simulink model "SchemaNO_DIS"  (R2020b)
settings: Solver=VariableStepAuto  StartTime=0.0  StopTime=20.0  RelTol=1e-3
undefined symbols (not defined in the file or in its folder): DELTA, G, U, Y
settings Model: Creator=teora  LastModifiedBy=teora

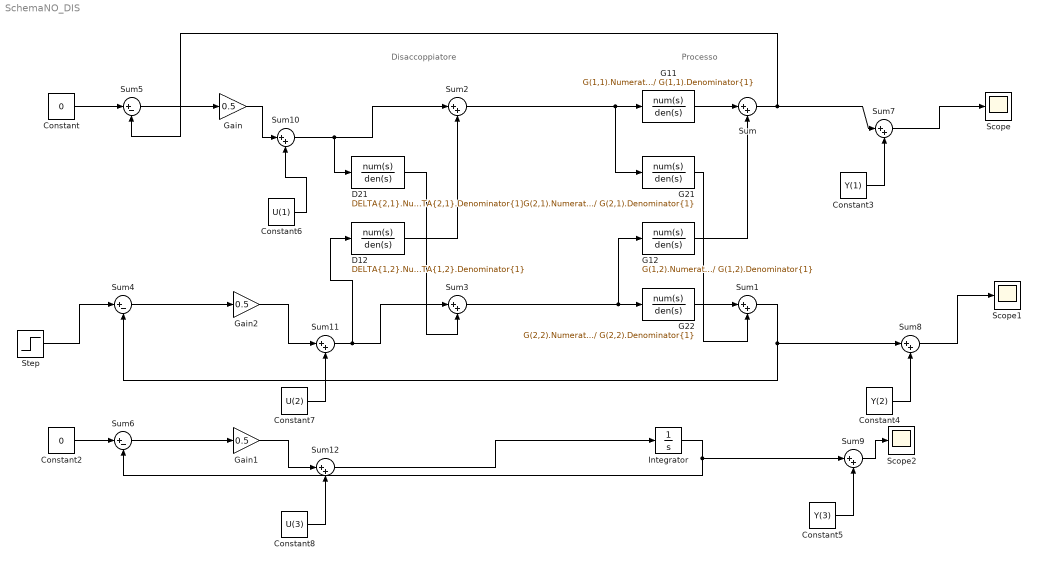
== system SchemaNO_DIS ==
  note: Disaccoppiatore
  note: Processo
  Constant : Constant  Value=0
  Constant2 : Constant  Value=0
  Constant3 : Constant  Value=Y(1)
  Constant4 : Constant  Value=Y(2)
  Constant5 : Constant  Value=Y(3)
  Constant6 : Constant  Value=U(1)
  Constant7 : Constant  Value=U(2)
  Constant8 : Constant  Value=U(3)
  D12 : TransferFcn  Numerator=DELTA{1,2}.Numerator{1}  Denominator=DELTA{1,2}.Denominator{1}
  D21 : TransferFcn  Numerator=DELTA{2,1}.Numerator{1}  Denominator=DELTA{2,1}.Denominator{1}
  G11 : TransferFcn  Numerator=G(1,1).Numerator{1}  Denominator=G(1,1).Denominator{1}
  G12 : TransferFcn  Numerator=G(1,2).Numerator{1}  Denominator=G(1,2).Denominator{1}
  G21 : TransferFcn  Numerator=G(2,1).Numerator{1}  Denominator=G(2,1).Denominator{1}
  G22 : TransferFcn  Numerator=G(2,2).Numerator{1}  Denominator=G(2,2).Denominator{1}
  Gain : Gain  Gain=0.5
  Gain1 : Gain  Gain=0.5
  Gain2 : Gain  Gain=0.5
  Integrator : Integrator
  Scope : Scope
  Scope1 : Scope
  Scope2 : Scope
  Step : Step  Time=5  After=67  SampleTime=0
  Sum{,1..3,7..12} (10 alike) : Sum  Inputs=|++
  Sum4 : Sum  Inputs=|+-
  Sum5 : Sum  Inputs=|+-
  Sum6 : Sum  Inputs=|+-
  wires:
  G11/1 -> Sum/1
  G22/1 -> Sum1/1
  G12/1 -> Sum/2
  G21/1 -> Sum1/2
  D21/1 -> Sum3/2
  D12/1 -> Sum2/2
  Sum2/1 -> G21/1, G11/1
  Sum3/1 -> G12/1, G22/1
  Step/1 -> Sum4/1
  Sum4/1 -> Gain2/1
  Sum1/1 -> Sum8/1, Sum4/2
  Constant/1 -> Sum5/1
  Sum/1 -> Sum7/1, Sum5/2
  Sum5/1 -> Gain/1
  Constant2/1 -> Sum6/1
  Sum6/1 -> Gain1/1
  Integrator/1 -> Sum9/1, Sum6/2
  Constant3/1 -> Sum7/2
  Sum7/1 -> Scope/1
  Constant4/1 -> Sum8/2
  Sum8/1 -> Scope1/1
  Constant5/1 -> Sum9/2
  Sum9/1 -> Scope2/1
  Constant6/1 -> Sum10/2
  Constant7/1 -> Sum11/2
  Constant8/1 -> Sum12/2
  Sum10/1 -> D21/1, Sum2/1
  Gain/1 -> Sum10/1
  Sum11/1 -> D12/1, Sum3/1
  Gain2/1 -> Sum11/1
  Sum12/1 -> Integrator/1
  Gain1/1 -> Sum12/1
